simulink model "CM670A_HwAg1Meas"  (R2013b)
settings: Solver=FixedStepDiscrete  SolverMode=SingleTasking  StartTime=0.0  StopTime=22  FixedStep=0.002  RelTol=1e-3
values from neighbouring files (symbols this model uses):
  ELECGLBPRM_DEGPERREV_DEGPERREV_F32 = DataDict.Constant    [CM670A_HwAg1Meas_DataDict.m]
  ELECGLBPRM_HWAGCENTROFFS_HWDEG_F32 = DataDict.Constant    [CM670A_HwAg1Meas_DataDict.m]
  ELECGLBPRM_HWAGSATNLOWRLIM_HWDEG_F32 = DataDict.Constant    [CM670A_HwAg1Meas_DataDict.m]
  ELECGLBPRM_HWAGSATNUPPRLIM_HWDEG_F32 = DataDict.Constant    [CM670A_HwAg1Meas_DataDict.m]
  ELECGLBPRM_HWAGSCA_ULS_F32 = DataDict.Constant    [CM670A_HwAg1Meas_DataDict.m]
  ELECGLBPRM_HWAGSPURGEARRAT_ULS_F32 = DataDict.Constant    [CM670A_HwAg1Meas_DataDict.m]
  ELECGLBPRM_HWAGSPURTORINGGEARRATSNSR0_ULS_F32 = DataDict.Constant    [CM670A_HwAg1Meas_DataDict.m]
  ELECGLBPRM_HWAGSPURTORINGGEARRATSNSR1_ULS_F32 = DataDict.Constant    [CM670A_HwAg1Meas_DataDict.m]
  ELECGLBPRM_NOFLT_CNT_U08 = DataDict.Constant    [CM670A_HwAg1Meas_DataDict.m]
  ELECGLBPRM_OFFSTRIMNOTPRFMD_CNT_U08 = DataDict.Constant    [CM670A_HwAg1Meas_DataDict.m]
  ELECGLBPRM_PRTCLFLT_CNT_U08 = DataDict.Constant    [CM670A_HwAg1Meas_DataDict.m]
  ELECGLBPRM_SKIPSTEPFLT_CNT_U08 = DataDict.Constant    [CM670A_HwAg1Meas_DataDict.m]
  ELECGLBPRM_SNSRINTFLT_CNT_U08 = DataDict.Constant    [CM670A_HwAg1Meas_DataDict.m]
  ELECGLBPRM_VRNRERRFLT_CNT_U08 = DataDict.Constant    [CM670A_HwAg1Meas_DataDict.m]
  HWAG10THTOOTHTRIG_CNT_U08 = DataDict.ConfigParam    [CM670A_HwAg1Meas_DataDict.m]
  HWAG11THTOOTHTRIG_CNT_U08 = DataDict.ConfigParam    [CM670A_HwAg1Meas_DataDict.m]
  HwAg1IfFlt = DataDict.NTC    [CM670A_HwAg1Meas_DataDict.m]
  HwAg1MeasHwAg1IfFltFailStep = DataDict.Calibration    [CM670A_HwAg1Meas_DataDict.m]
  HwAg1MeasHwAg1IfFltPassStep = DataDict.Calibration    [CM670A_HwAg1Meas_DataDict.m]
  HwAg1MeasHwAg1Snsr0PrtclFltFailStep = DataDict.Calibration    [CM670A_HwAg1Meas_DataDict.m]
  HwAg1MeasHwAg1Snsr0PrtclFltPassStep = DataDict.Calibration    [CM670A_HwAg1Meas_DataDict.m]
  HwAg1MeasHwAg1Snsr1PrtclFltFailStep = DataDict.Calibration    [CM670A_HwAg1Meas_DataDict.m]
  HwAg1MeasHwAg1Snsr1PrtclFltPassStep = DataDict.Calibration    [CM670A_HwAg1Meas_DataDict.m]
  HwAg1MeasSnsr0Rev = DataDict.Calibration    [CM670A_HwAg1Meas_DataDict.m]
  HwAg1MeasSnsr1Rev = DataDict.Calibration    [CM670A_HwAg1Meas_DataDict.m]
  HwAg1MeasStep = DataDict.Calibration    [CM670A_HwAg1Meas_DataDict.m]
  HwAg1MeasVrnrErrThd = DataDict.Calibration    [CM670A_HwAg1Meas_DataDict.m]
  HwAg1MfgFlt = DataDict.NTC    [CM670A_HwAg1Meas_DataDict.m]
  HwAg1Snsr0PrtclFlt = DataDict.NTC    [CM670A_HwAg1Meas_DataDict.m]
  HwAg1Snsr1PrtclFlt = DataDict.NTC    [CM670A_HwAg1Meas_DataDict.m]
undefined symbols (not defined in the file or in its folder): NtcSts1, sigbuilder_block, SigQlfr1
libraries: simulink x30, NxtrNvM x3
(part 1 of 5)
settings Model: CovMetricSettings=dcmtrzoiw  CovFilter=CM670A_HwAg1Meas_covfilter  CovHTMLOptions=-sRT=1 -aTS=1 -bRG=1 -bTC=1 -hTR=0 -nFC=0 -scm=1 -bcm=1 -xEv=0  CovModelRefEnable=off  Creator=CZ68DS  LastModifiedBy=CZ68DS
settings SolverCC: PositivePriorityOrder=on  AutoInsertRateTranBlk=on  InsertRTBMode=Always
settings DataIOCC: LimitDataPoints=off  SaveFormat=Structure  ReturnWorkspaceOutputs=on
settings OptimizationCC: InlineParams=on  InlineInvariantSignals=on  PassReuseOutputArgsAs=Individual arguments  ZeroExternalMemoryAtStartup=off  ZeroInternalMemoryAtStartup=off  EfficientFloat2IntCast=on  OptimizeModelRefInitCode=on  LifeSpan=1
settings DebuggingCC: SignalInfNanChecking=error  ReadBeforeWriteMsg=EnableAllAsWarning  WriteAfterWriteMsg=EnableAllAsWarning  WriteAfterReadMsg=EnableAllAsWarning  UnderspecifiedInitializationDetection=Simplified  MergeDetectMultiDrivingBlocksExec=error  SolverPrmCheckMsg=error  InheritedTsInSrcMsg=error  MultiTaskDSMMsg=warning  SingleTaskRateTransMsg=error  TasksWithSamePriorityMsg=error  SigSpecEnsureSampleTimeMsg=error  CheckMatrixSingularityMsg=error  ParameterUnderflowMsg=error  ParameterPrecisionLossMsg=error  ParameterTunabilityLossMsg=error  FixptConstUnderflowMsg=warning  FixptConstOverflowMsg=warning  FixptConstPrecisionLossMsg=warning  VectorMatrixConversionMsg=error  SignalLabelMismatchMsg=error  UnconnectedInputMsg=error  UnconnectedOutputMsg=error  UnconnectedLineMsg=error  SFcnCompatibilityMsg=error  FrameProcessingCompatibilityMsg=error  UniqueDataStoreMsg=warning  BusObjectLabelMismatch=error  RootOutportRequireBusObject=error  AssertControl=DisableAll  ModelReferenceIOMsg=error  ModelReferenceVersionMismatchMessage=warning  ModelReferenceIOMismatchMessage=error  ModelReferenceDataLoggingMessage=error  StateNameClashWarn=warning  StrictBusMsg=ErrorOnBusTreatedAsVector  NonBusSignalsTreatedAsBus=error  SFUnexpectedBacktrackingDiag=error  SFInvalidInputDataAccessInChartInitDiag=error  SFNoUnconditionalDefaultTransitionDiag=error  SFTransitionOutsideNaturalParentDiag=error  SFUnconditionalTransitionShadowingDiag=error  SFUndirectedBroadcastEventsDiag=error
settings HardwareCC: ProdEndianess=LittleEndian  ProdHWDeviceType=Texas Instruments->TMS470
settings ModelReferenceCC: ModelReferenceNumInstancesAllowed=Single
settings RTWCC: SystemTargetFile=autosar.tlc  GenCodeOnly=on  TemplateMakefile=ert_default_tmf  Description=AUTOSAR  GenerateReport=on  ProcessScript=autosar_make_rtw_hook  LaunchReport=on
settings CodeAppCC: GenerateComments=off  IgnoreCustomStorageClasses=off  IgnoreTestpoints=on  CustomSymbolStrType=$N$R$M  CustomSymbolStrBlkIO=$N$M  SimulinkBlockComments=off
settings STFCustomTargetCC: CodeReplacementLibrary=C89/C90 (ANSI)  ParMdlRefBuildCompliant=on  CompOptLevelCompliant=on  IncludeMdlTerminateFcn=off  CombineOutputUpdateFcns=on  SuppressErrorStatus=on  ERTFirstTimeCompliant=on  ERTCustomFileBanners=on  SupportNonFinite=off  SupportComplex=off  SupportContinuousTime=off  SupportNonInlinedSFcns=off  MATLABClassNameForMDSCustomization=Simulink.SoftwareTarget.ERTCustomization  AutosarCompliant=on  GRTInterface=off  SystemTargetFile=autosar.tlc
settings ERTTargetCC: CodeReplacementLibrary=C89/C90 (ANSI)  ConcurrentExecutionCompliant=off  IncludeMdlTerminateFcn=off  SuppressErrorStatus=on  SupportNonFinite=off  SupportComplex=off  ModelStepFunctionPrototypeControlCompliant=off  CPPClassGenCompliant=off  AutosarCompliant=on  InlinedParameterPlacement=NonHierarchical  ERTCustomFileTemplate=example_file_process.tlc  EnableUserReplacementTypes=on

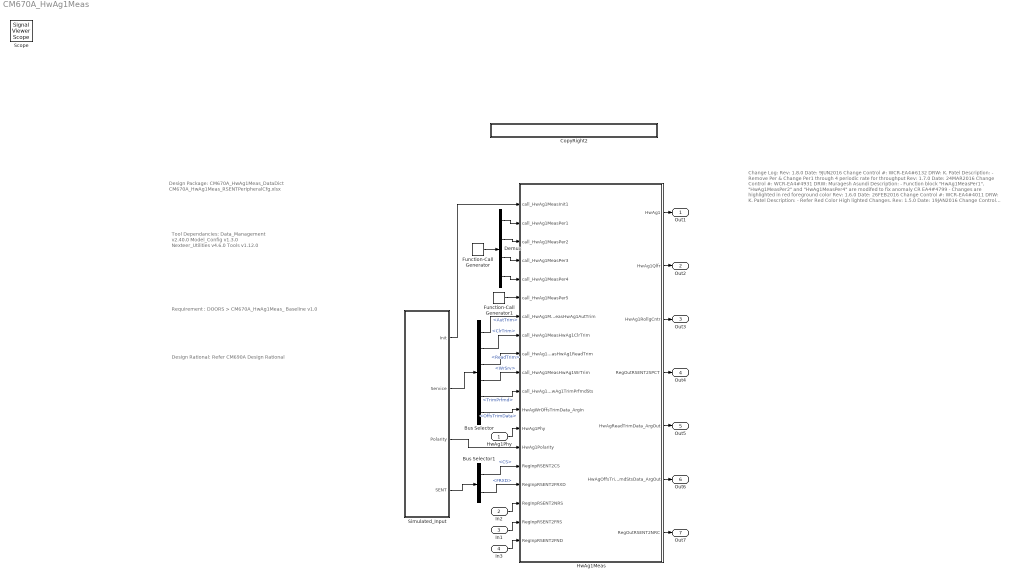
== system CM670A_HwAg1Meas ==
  note: Tool Dependancies:
      |
      | Data_Management v2.40.0
      | Model_Config v1.3.0
      | Nexteer_Utilities v4.6.0
      | Tools v1.12.0
  note: Design Package:
      |
      | CM670A_HwAg1Meas_DataDict
      | CM670A_HwAg1Meas_RSENTPeripheralCfg.xlsx
  note: Requirement :
      |
      | DOORS > CM670A_HwAg1Meas_ Baseline v1.0
  note: Change Log:
      |
      | Rev: 1.8.0
      | Date: 9JUN2016
      | Change Control #: WCR-EA4#6132
      | DRW: K. Patel
      | Description:
      | - Remove Per & Change Per1 through 4 periodic rate for throughput
      |
      |
      | Rev: 1.7.0
      | Date: 24MAR2016
      | Change Control #: WCR-EA4#4931
      | DRW: Muragesh Asundi
      | Description:
      | - Function block "HwAg1MeasPer1", "HwAg1MeasPer2" and "HwAg1MeasPer4" are modifed
      |   to fix anomaly CR EA4#4799
      | - Changes are highlighted in red foreground color
      |
      | Rev: 1.6.0
      | Date: 26FEB2016
      | Change Control #: WCR-EA4#4011
      | DRW: K. Patel
      | Description:
      | - Refer Red Color High lighted Changes.
      |
      | Rev: 1.5.0
      | Date: 19JAN2016
      | Change Control #: WCR-EA4#3382
      | DRW: K. Patel
      | Description:
      | - Refer Red Color High lighted Changes.
      | - "CM670A_HwAg1Meas_RSENTPeripheralCfg.xlsx" change
      | - m file change
      |
      | Rev: 1.4.0
      | Date: 02DEC2015
      | Change Control #: WCR-EA4#2679 Anomaly Fix
      | DRW: K. Patel
      | Description:
      | - Refer Red Color High lighted Changes.
      |
      | Rev: 1.3.0
      | Date: 06OCT2015
      | Change Control #: WCR-EA4#1873, Anomaly:EA4#1856
      | DRW: K. Patel
      | Description:
      | - Skip step Interface fault
      |
      | Rev: 1.2.0
      | Date: 8SEPT2015
      | Change Control #: WCR-EA4#1530, Anomaly:EA4#1354, Anomaly:EA4#1508
      | DRW: K. Patel
      | Description:
      | - Reading Nibble Fix (peripheral register configuration change)
      | - Cleaning CS register before SPCT
      | - Sensor Synchronization logic added
      |
      | Rev: 1.1.0
      | Date: 11AUG2015
      | Change Control #: WCR-EA4#1271
      | DRW: K. Patel
      | Description:
      | - M file correction & Model Correction
      |
      | Rev: 1.0.0
      | Date: 23JUN2015
      | Change Control #: WCR-EA4#910
      | DRW: K. Patel
      | Description:
      | - Initial Release
      |
      | DRW: Keyur Patel
      | Scope:
      | - Model intent to implement EA4 SENT2 based Digital HandWheel Angle implementation for T1xx.
      |    model runs at different function rate:
      |       1) Init - Configure Peripheral
      |       2) 4ms - Per1 & Per2 use for SENT Trigger
      |       3) 4ms - Per3 Read SENT Data from 10 Tooth & Protocol Fault
      |       4) 4ms - Per4 Read SENT Data from 11 Tooth & Protocol Fault
      |       5) 4ms - Per5 Final HwAg calculation
      |       6) 100ms - Per6 Trim Not Performed evaluation
      |       7) Event Trim Service - Auto, Clear, Write, Read, Trim Performed Status
      | - Copyright Blocks added to each layer
  note: Design Rational:
      |
      | Refer CM690A Design Rational
  HwAg1Phy : Inport
  In2 : Inport  Port=2
  In1 : Inport  Port=3
  In3 : Inport  Port=4
  Bus Selector : BusSelector  OutputSignals=AutTrim,ClrTrim,ReadTrim,WrSrv,TrimPrfmd,OffsTrimData
  Bus Selector1 : BusSelector  OutputSignals=CS,FRXD
  CopyRight2 : Subsystem  Description=|  mask(Copyright Information){none=on}
      | Copyright info block.                                               
      |                                                                     
      | Place copyright information at the top of every subsystem in design.
      mask prompts: none "No parameters"
      mask help: Place copyright information at the top of every subsystem in design.
      mask Display:
      | NxtrConf = 'Nexteer Confidential';
      | 
      | sys = bdroot; %handle for the current model ("system")
      | first = get_param(sys,'Created');
      | first = first(end-3:end);  %year is last four digits
      | 
      | last = get_param(sys,'LastModifiedDate');
      | if isempty(last)
      |     last = datestr(now,'yyyy');
      | else
      |     last = last(end-3:end);
      | end
      | 
      | if strcmp(first,last)
      |     fprintf('%s -- Copyright %s Nexteer',NxtrConf,first)
      | else
      |     fprintf('%s -- %s%s- %s Nexteer',NxtrConf,char(169),first,last)
      | end
  Demux : Demux
  Function-Call Generator : simulink/Ports & Subsystems/Function-Call Generator  sample_time=0.002  numberOfIterations=1
      settings: AttributesFormatString=%<sample_time>
  Function-Call Generator1 : simulink/Ports & Subsystems/Function-Call Generator  sample_time=0.100  numberOfIterations=1
  HwAg1Meas : Subsystem  RequirementInfo={} %GIDa_1b511019_32d3_4208_ad3f_5416ab2f5672
  Simulated_Input : Subsystem  Description=Do not Code this block
      settings: AttributesFormatString=%<Description>
  Out1 : Outport
  Out2 : Outport  Port=2
  Out3 : Outport  Port=3
  Out4 : Outport  Port=4
  Out5 : Outport  Port=5
  Out6 : Outport  Port=6
  Out7 : Outport  Port=7
  Scope : SignalViewerScope  IOType=viewer  SampleTime=-1  RefreshTime=0.035000
      settings: YMin=-10  YMax=10
  wires:
  Function-Call Generator/1 -> Demux/1
  HwAg1Meas/1(HwAg1) -> Out1/1
  Demux/1 -> HwAg1Meas/2(call_HwAg1MeasPer1)
  Demux/2 -> HwAg1Meas/3(call_HwAg1MeasPer2)
  Demux/3 -> HwAg1Meas/4(call_HwAg1MeasPer3)
  Function-Call Generator1/1 -> HwAg1Meas/6(call_HwAg1MeasPer5)
  Simulated_Input/3(Polarity) -> HwAg1Meas/14(HwAg1Polarity)
  HwAg1Meas/2(HwAg1Qlfr) -> Out2/1
  HwAg1Meas/3(HwAg1RollgCntr) -> Out3/1
  HwAg1Meas/4(RegOutRSENT2SPCT) -> Out4/1
  HwAg1Meas/5(HwAgReadTrimData_ArgOut) -> Out5/1
  HwAg1Meas/6(HwAgOffsTrimPrfmdStsData_ArgOut) -> Out6/1
  Simulated_Input/2(Service) -> Bus Selector/1
  Bus Selector/1 -> HwAg1Meas/7(call_HwAg1MeasHwAg1AutTrim)  "<AutTrim>"
  Bus Selector/2 -> HwAg1Meas/8(call_HwAg1MeasHwAg1ClrTrim)  "<ClrTrim>"
  Bus Selector/3 -> HwAg1Meas/9(call_HwAg1MeasHwAg1ReadTrim)  "<ReadTrim>"
  Bus Selector/4 -> HwAg1Meas/10(call_HwAg1MeasHwAg1WrTrim)  "<WrSrv>"
  Bus Selector/5 -> HwAg1Meas/11(call_HwAg1MeasHwAg1TrimPrfmdSts)  "<TrimPrfmd>"
  Bus Selector/6 -> HwAg1Meas/12(HwAgWrOffsTrimData_ArgIn)  "<OffsTrimData>"
  Simulated_Input/1(Init) -> HwAg1Meas/1(call_HwAg1MeasInit1)
  HwAg1Phy/1 -> HwAg1Meas/13(HwAg1Phy)
  Simulated_Input/4(SENT) -> Bus Selector1/1
  Bus Selector1/1 -> HwAg1Meas/15(RegInpRSENT2CS)  "<CS>"
  Bus Selector1/2 -> HwAg1Meas/16(RegInpRSENT2FRXD)  "<FRXD>"
  In2/1 -> HwAg1Meas/17(RegInpRSENT2NRS)
  HwAg1Meas/7(RegOutRSENT2NRC) -> Out7/1
  In1/1 -> HwAg1Meas/18(RegInpRSENT2FRS)
  In3/1 -> HwAg1Meas/19(RegInpRSENT2FND)
  Demux/4 -> HwAg1Meas/5(call_HwAg1MeasPer4)

== system CM670A_HwAg1Meas/CopyRight2 ==

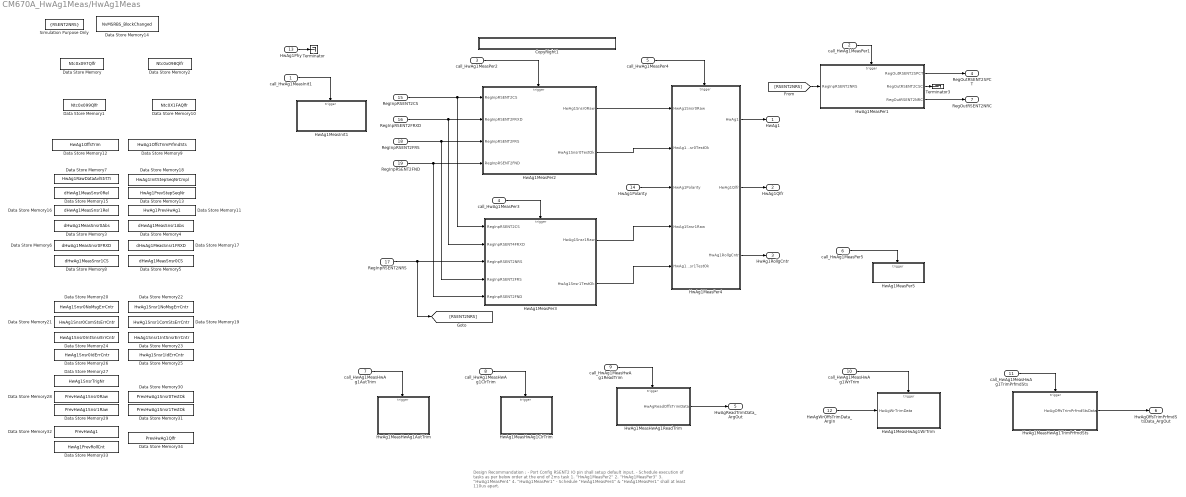
== system CM670A_HwAg1Meas/HwAg1Meas ==
  note: Design Recommandation :
      |
      | - Port Config RSENT2 IO pin shall setup default input.
      | - Schedule execution of tasks as per below order at the end of 2ms task
      |
      |    1.  "HwAg1MeasPer2"
      |    2.  "HwAg1MeasPer3"
      |    3.  "HwAg1MeasPer4"
      |    4.  "HwAg1MeasPer1"
      |
      | - Schedule  "HwAg1MeasPer4" & "HwAg1MeasPer1"  shall at least 110us apart.
  call_HwAg1MeasInit1 : Inport
  call_HwAg1MeasPer1 : Inport  Port=2
      settings: AttributesFormatString=%<SampleTime>
  call_HwAg1MeasPer2 : Inport  Port=3
      settings: AttributesFormatString=%<SampleTime>
  call_HwAg1MeasPer3 : Inport  Port=4
      settings: AttributesFormatString=%<SampleTime>
  call_HwAg1MeasPer4 : Inport  Description=4ms  Port=5
      settings: AttributesFormatString=%<SampleTime>
  call_HwAg1MeasPer5 : Inport  Description=100ms  Port=6
      settings: AttributesFormatString=%<Description>
  call_HwAg1MeasHwAg1AutTrim : Inport  Description=Event  Port=7
      settings: AttributesFormatString=%<Description>
  call_HwAg1MeasHwAg1ClrTrim : Inport  Description=Event  Port=8
      settings: AttributesFormatString=%<Description>
  call_HwAg1MeasHwAg1ReadTrim : Inport  Description=Event  Port=9
      settings: AttributesFormatString=%<Description>
  call_HwAg1MeasHwAg1WrTrim : Inport  Description=Event  Port=10
      settings: AttributesFormatString=%<Description>
  call_HwAg1MeasHwAg1TrimPrfmdSts : Inport  Description=Event  Port=11
      settings: AttributesFormatString=%<Description>
  HwAgWrOffsTrimData_ArgIn : Inport  Port=12
  HwAg1Phy : Inport  Port=13
  HwAg1Polarity : Inport  Port=14  OutDataTypeStr=int8
  RegInpRSENT2CS : Inport  Port=15
  RegInpRSENT2FRXD : Inport  Port=16
  RegInpRSENT2NRS : Inport  Port=17
  RegInpRSENT2FRS : Inport  Port=18
  RegInpRSENT2FND : Inport  Port=19
  CopyRight1 : Subsystem  Description=|  mask(Copyright Information){none=on}
      | Copyright info block.                                               
      |                                                                     
      | Place copyright information at the top of every subsystem in design.
      mask prompts: none "No parameters"
      mask help: Place copyright information at the top of every subsystem in design.
      mask Display:
      | NxtrConf = 'Nexteer Confidential';
      | 
      | sys = bdroot; %handle for the current model ("system")
      | first = get_param(sys,'Created');
      | first = first(end-3:end);  %year is last four digits
      | 
      | last = get_param(sys,'LastModifiedDate');
      | if isempty(last)
      |     last = datestr(now,'yyyy');
      | else
      |     last = last(end-3:end);
      | end
      | 
      | if strcmp(first,last)
      |     fprintf('%s -- Copyright %s Nexteer',NxtrConf,first)
      | else
      |     fprintf('%s -- %s%s- %s Nexteer',NxtrConf,char(169),first,last)
      | end
  Data Store Memory11 : DataStoreMemory  DataStoreName=HwAg1PrevHwAg1  ReadBeforeWriteMsg=warning  WriteAfterWriteMsg=warning  WriteAfterReadMsg=warning  StateMustResolveToSignalObject=on
  Data Store Memory12 : DataStoreMemory  DataStoreName=HwAg1OffsTrim  ReadBeforeWriteMsg=warning  WriteAfterWriteMsg=warning  WriteAfterReadMsg=warning
  Data Store Memory13 : DataStoreMemory  DataStoreName=HwAg1PrevStepSeqNr  ReadBeforeWriteMsg=warning  WriteAfterWriteMsg=warning  WriteAfterReadMsg=warning  StateMustResolveToSignalObject=on
  Data Store Memory14 : DataStoreMemory  Description=|  DataStoreName=NvMSRBS_BlockChanged  ReadBeforeWriteMsg=warning  WriteAfterWriteMsg=warning  WriteAfterReadMsg=warning
      | Simulation Purpose Only.
      | Do Not Code this block
      | NVM Manager Owns this requirement
      settings: AttributesFormatString=%<Description>
  Data Store Memory15 : DataStoreMemory  DataStoreName=dHwAg1MeasSnsr0Rel  ReadBeforeWriteMsg=warning  WriteAfterWriteMsg=warning  WriteAfterReadMsg=warning  StateMustResolveToSignalObject=on
  Data Store Memory16 : DataStoreMemory  DataStoreName=dHwAg1MeasSnsr1Rel  ReadBeforeWriteMsg=warning  WriteAfterWriteMsg=warning  WriteAfterReadMsg=warning  StateMustResolveToSignalObject=on
  Data Store Memory17 : DataStoreMemory  DataStoreName=dHwAg1MeasSnsr1FRXD  ReadBeforeWriteMsg=warning  WriteAfterWriteMsg=warning  WriteAfterReadMsg=warning  StateMustResolveToSignalObject=on
  Data Store Memory18 : DataStoreMemory  DataStoreName=HwAg1InitStepSeqNrCmpl  ReadBeforeWriteMsg=warning  WriteAfterWriteMsg=warning  WriteAfterReadMsg=warning  StateMustResolveToSignalObject=on
  Data Store Memory19 : DataStoreMemory  DataStoreName=HwAg1Snsr1ComStsErrCntr  ReadBeforeWriteMsg=warning  WriteAfterWriteMsg=warning  WriteAfterReadMsg=warning  StateMustResolveToSignalObject=on
  Data Store Memory20 : DataStoreMemory  DataStoreName=HwAg1Snsr0NoMsgErrCntr  ReadBeforeWriteMsg=warning  WriteAfterWriteMsg=warning  WriteAfterReadMsg=warning  StateMustResolveToSignalObject=on
  Data Store Memory21 : DataStoreMemory  DataStoreName=HwAg1Snsr0ComStsErrCntr  ReadBeforeWriteMsg=warning  WriteAfterWriteMsg=warning  WriteAfterReadMsg=warning  StateMustResolveToSignalObject=on
  Data Store Memory22 : DataStoreMemory  DataStoreName=HwAg1Snsr1NoMsgErrCntr  ReadBeforeWriteMsg=warning  WriteAfterWriteMsg=warning  WriteAfterReadMsg=warning  StateMustResolveToSignalObject=on
  Data Store Memory23 : DataStoreMemory  DataStoreName=HwAg1Snsr1IntSnsrErrCntr  ReadBeforeWriteMsg=warning  WriteAfterWriteMsg=warning  WriteAfterReadMsg=warning  StateMustResolveToSignalObject=on
  Data Store Memory24 : DataStoreMemory  DataStoreName=HwAg1Snsr0IntSnsrErrCntr  ReadBeforeWriteMsg=warning  WriteAfterWriteMsg=warning  WriteAfterReadMsg=warning  StateMustResolveToSignalObject=on
  Data Store Memory25 : DataStoreMemory  DataStoreName=HwAg1Snsr1IdErrCntr  ReadBeforeWriteMsg=warning  WriteAfterWriteMsg=warning  WriteAfterReadMsg=warning  StateMustResolveToSignalObject=on
  Data Store Memory26 : DataStoreMemory  DataStoreName=HwAg1Snsr0IdErrCntr  ReadBeforeWriteMsg=warning  WriteAfterWriteMsg=warning  WriteAfterReadMsg=warning  StateMustResolveToSignalObject=on
  Data Store Memory27 : DataStoreMemory  DataStoreName=HwAg1SnsrTrigNr  ReadBeforeWriteMsg=warning  WriteAfterWriteMsg=warning  WriteAfterReadMsg=warning  StateMustResolveToSignalObject=on
  Data Store Memory28 : DataStoreMemory  DataStoreName=PrevHwAg1Snsr0Raw  ReadBeforeWriteMsg=warning  WriteAfterWriteMsg=warning  WriteAfterReadMsg=warning  StateMustResolveToSignalObject=on
  Data Store Memory29 : DataStoreMemory  DataStoreName=PrevHwAg1Snsr1Raw  ReadBeforeWriteMsg=warning  WriteAfterWriteMsg=warning  WriteAfterReadMsg=warning  StateMustResolveToSignalObject=on
  Data Store Memory3 : DataStoreMemory  DataStoreName=dHwAg1MeasSnsr0Abs  ReadBeforeWriteMsg=warning  WriteAfterWriteMsg=warning  WriteAfterReadMsg=warning  StateMustResolveToSignalObject=on
  Data Store Memory30 : DataStoreMemory  DataStoreName=PrevHwAg1Snsr0TestOk  ReadBeforeWriteMsg=warning  WriteAfterWriteMsg=warning  WriteAfterReadMsg=warning  StateMustResolveToSignalObject=on
  Data Store Memory31 : DataStoreMemory  DataStoreName=PrevHwAg1Snsr1TestOk  ReadBeforeWriteMsg=warning  WriteAfterWriteMsg=warning  WriteAfterReadMsg=warning  StateMustResolveToSignalObject=on
  Data Store Memory32 : DataStoreMemory  DataStoreName=PrevHwAg1  ReadBeforeWriteMsg=warning  WriteAfterWriteMsg=warning  WriteAfterReadMsg=warning  StateMustResolveToSignalObject=on
  Data Store Memory33 : DataStoreMemory  DataStoreName=HwAg1PrevRollCnt  ReadBeforeWriteMsg=warning  WriteAfterWriteMsg=warning  WriteAfterReadMsg=warning  StateMustResolveToSignalObject=on
  Data Store Memory34 : DataStoreMemory  DataStoreName=PrevHwAg1Qlfr  ReadBeforeWriteMsg=warning  WriteAfterWriteMsg=warning  WriteAfterReadMsg=warning  InitialValue=SigQlfr1.SIGQLFR_NORES  OutDataTypeStr=Enum: SigQlfr1  StateMustResolveToSignalObject=on
  Data Store Memory4 : DataStoreMemory  DataStoreName=dHwAg1MeasSnsr1Abs  ReadBeforeWriteMsg=warning  WriteAfterWriteMsg=warning  WriteAfterReadMsg=warning  StateMustResolveToSignalObject=on
  Data Store Memory5 : DataStoreMemory  DataStoreName=dHwAg1MeasSnsr0CS  ReadBeforeWriteMsg=warning  WriteAfterWriteMsg=warning  WriteAfterReadMsg=warning  StateMustResolveToSignalObject=on
  Data Store Memory6 : DataStoreMemory  DataStoreName=dHwAg1MeasSnsr0FRXD  ReadBeforeWriteMsg=warning  WriteAfterWriteMsg=warning  WriteAfterReadMsg=warning  StateMustResolveToSignalObject=on
  Data Store Memory7 : DataStoreMemory  DataStoreName=HwAg1RawDataAvlStrtTi  ReadBeforeWriteMsg=warning  WriteAfterWriteMsg=warning  WriteAfterReadMsg=warning  StateMustResolveToSignalObject=on
  Data Store Memory8 : DataStoreMemory  DataStoreName=dHwAg1MeasSnsr1CS  ReadBeforeWriteMsg=warning  WriteAfterWriteMsg=warning  WriteAfterReadMsg=warning  StateMustResolveToSignalObject=on
  Data Store Memory9 : DataStoreMemory  DataStoreName=HwAg1OffsTrimPrfmdSts  ReadBeforeWriteMsg=warning  WriteAfterWriteMsg=warning  WriteAfterReadMsg=warning
  Data Store Memory : DataStoreMemory  DataStoreName=Ntc0x097Qlfr  ReadBeforeWriteMsg=warning  WriteAfterWriteMsg=warning  WriteAfterReadMsg=warning  OutDataTypeStr=uint8
      settings: AttributesFormatString=|
      | Simulation Purpose Only.
      | Do Not Code this block
      | Diagnostic Manager Owns this requirement
  Data Store Memory1 : DataStoreMemory  DataStoreName=Ntc0x099Qlfr  ReadBeforeWriteMsg=warning  WriteAfterWriteMsg=warning  WriteAfterReadMsg=warning  OutDataTypeStr=uint8
      settings: AttributesFormatString=|
      | Simulation Purpose Only.
      | Do Not Code this block
      | Diagnostic Manager Owns this requirement
  Data Store Memory10 : DataStoreMemory  DataStoreName=Ntc0X1FAQlfr  ReadBeforeWriteMsg=warning  WriteAfterWriteMsg=warning  WriteAfterReadMsg=warning  OutDataTypeStr=uint8
      settings: AttributesFormatString=|
      | Simulation Purpose Only.
      | Do Not Code this block
      | Diagnostic Manager Owns this requirement
  Data Store Memory2 : DataStoreMemory  DataStoreName=Ntc0x098Qlfr  ReadBeforeWriteMsg=warning  WriteAfterWriteMsg=warning  WriteAfterReadMsg=warning  OutDataTypeStr=uint8
      settings: AttributesFormatString=|
      | Simulation Purpose Only.
      | Do Not Code this block
      | Diagnostic Manager Owns this requirement
  HwAg1MeasHwAg1AutTrim : Subsystem  RequirementInfo={'linktype_rmi_doors' '0000cf44 (/ESG Group/FDD Module Requirements/EA4 Specific/CM670A_HwAg1Meas)' '#CM670A_90' 'true' 'REQ: CM670A_90' '' } %GIDa_ea94ffee_6a60_4ad4_8777_fa2e1209d3e2  TreatAsAtomicUnit=on
  HwAg1MeasHwAg1ClrTrim : Subsystem  RequirementInfo={'linktype_rmi_doors' '0000cf44 (/ESG Group/FDD Module Requirements/EA4 Specific/CM670A_HwAg1Meas)' '#CM670A_88' 'true' 'REQ: CM670A_88' '' } %GIDa_ac4d7135_c09e_4b99_819a_ee37d51d6394  TreatAsAtomicUnit=on
  HwAg1MeasHwAg1ReadTrim : Subsystem  RequirementInfo={'linktype_rmi_doors' '0000cf44 (/ESG Group/FDD Module Requirements/EA4 Specific/CM670A_HwAg1Meas)' '#CM670A_86' 'true' 'REQ: CM670A_86' '' } %GIDa_cdad271c_f4aa_4684_91af_0774478ab1dd  TreatAsAtomicUnit=on
  HwAg1MeasHwAg1TrimPrfmdSts : Subsystem  RequirementInfo={'linktype_rmi_doors' '0000cf44 (/ESG Group/FDD Module Requirements/EA4 Specific/CM670A_HwAg1Meas)' '#CM670A_87' 'true' 'REQ: CM670A_87' '' } %GIDa_f9e60140_9f20_40c9_8f6d_edf000506692  TreatAsAtomicUnit=on
  HwAg1MeasHwAg1WrTrim : Subsystem  RequirementInfo={'linktype_rmi_doors' '0000cf44 (/ESG Group/FDD Module Requirements/EA4 Specific/CM670A_HwAg1Meas)' '#CM670A_89' 'true' 'REQ: CM670A_89' '' } %GIDa_3e323fa6_2ebf_495c_adb5_a3e2347a88cc  TreatAsAtomicUnit=on
  HwAg1MeasInit1 : Subsystem  TreatAsAtomicUnit=on
  HwAg1MeasPer1 : Subsystem  RequirementInfo={'linktype_rmi_doors' '0000cf44 (/ESG Group/FDD Module Requirements/EA4 Specific/CM670A_HwAg1Meas)' '#CM670A_53' 'true' 'REQ: CM670A_53' '' } %GIDa_bc322e89_7505_4ced_bd58_d5630035f58c  TreatAsAtomicUnit=on
  HwAg1MeasPer2 : Subsystem  RequirementInfo={'linktype_rmi_doors' '0000cf44 (/ESG Group/FDD Module Requirements/EA4 Specific/CM670A_HwAg1Meas)' '#CM670A_54' 'true' 'REQ: CM670A_54' '' ; 'linktype_rmi_doors' '0000cf44 (/ESG Group/FDD Module Requirements/EA4 Specific/CM670A_HwAg1Meas)' '#CM670A_39' 'true' 'REQ: CM670A_39' '' } %GIDa_9b2c116c_3a4f_439a_af77_b112da5d765b  TreatAsAtomicUnit=on
  HwAg1MeasPer3 : Subsystem  RequirementInfo={'linktype_rmi_doors' '0000cf44 (/ESG Group/FDD Module Requirements/EA4 Specific/CM670A_HwAg1Meas)' '#CM670A_54' 'true' 'REQ: CM670A_54' '' ; 'linktype_rmi_doors' '0000cf44 (/ESG Group/FDD Module Requirements/EA4 Specific/CM670A_HwAg1Meas)' '#CM670A_60' 'true' 'REQ: CM670A_60' '' } %GIDa_7cda62b4_5588_448d_b03e_99bd27827f7d  TreatAsAtomicUnit=on
  HwAg1MeasPer4 : Subsystem  RequirementInfo={'linktype_rmi_doors' '0000cf44 (/ESG Group/FDD Module Requirements/EA4 Specific/CM670A_HwAg1Meas)' '#CM670A_95' 'true' 'REQ: CM670A_95' '' } %GIDa_d2359c71_dfd5_4281_9f6c_59b61df0ca5b  TreatAsAtomicUnit=on
  HwAg1MeasPer5 : Subsystem  RequirementInfo={'linktype_rmi_doors' '0000cf44 (/ESG Group/FDD Module Requirements/EA4 Specific/CM670A_HwAg1Meas)' '#CM670A_80' 'true' 'REQ: CM670A_80' '' } %GIDa_d0a6efa9_4f14_452b_9991_ec4ccddab763  TreatAsAtomicUnit=on
  Simulation Purpose Only : GotoTagVisibility  GotoTag=RSENT2NRS
  Terminator : Terminator
  Terminator3 : Terminator
  HwAg1 : Outport
  HwAg1Qlfr : Outport  Port=2
  HwAg1RollgCntr : Outport  Port=3
  RegOutRSENT2SPCT : Outport  Port=4
  HwAgReadTrimData_ArgOut : Outport  Port=5
  HwAgOffsTrimPrfmdStsData_ArgOut : Outport  Port=6
  RegOutRSENT2NRC : Outport  Port=7
  wires:
  call_HwAg1MeasPer2/1 -> HwAg1MeasPer2/Trigger
  call_HwAg1MeasInit1/1 -> HwAg1MeasInit1/Trigger
  RegInpRSENT2CS/1 -> HwAg1MeasPer3/1(RegInpRSENT2CS), HwAg1MeasPer2/1(RegInpRSENT2CS)
  HwAg1Phy/1 -> Terminator/1
  HwAg1MeasPer4/1(HwAg1) -> HwAg1/1
  HwAg1MeasPer4/2(HwAg1Qlfr) -> HwAg1Qlfr/1
  HwAg1MeasPer4/3(HwAg1RollgCntr) -> HwAg1RollgCntr/1
  call_HwAg1MeasPer3/1 -> HwAg1MeasPer3/Trigger
  call_HwAg1MeasPer4/1 -> HwAg1MeasPer4/Trigger
  HwAg1Polarity/1 -> HwAg1MeasPer4/3(HwAg1Polarity)
  call_HwAg1MeasPer1/1 -> HwAg1MeasPer1/Trigger
  call_HwAg1MeasHwAg1AutTrim/1 -> HwAg1MeasHwAg1AutTrim/Trigger
  call_HwAg1MeasHwAg1ClrTrim/1 -> HwAg1MeasHwAg1ClrTrim/Trigger
  call_HwAg1MeasHwAg1ReadTrim/1 -> HwAg1MeasHwAg1ReadTrim/Trigger
  call_HwAg1MeasHwAg1WrTrim/1 -> HwAg1MeasHwAg1WrTrim/Trigger
  call_HwAg1MeasHwAg1TrimPrfmdSts/1 -> HwAg1MeasHwAg1TrimPrfmdSts/Trigger
  HwAgWrOffsTrimData_ArgIn/1 -> HwAg1MeasHwAg1WrTrim/1(HwAgWrTrimData)
  HwAg1MeasHwAg1ReadTrim/1(HwAgReadOffsTrimData) -> HwAgReadTrimData_ArgOut/1
  HwAg1MeasHwAg1TrimPrfmdSts/1(HwAgOffsTrimPrfmdStsData) -> HwAgOffsTrimPrfmdStsData_ArgOut/1
  call_HwAg1MeasPer5/1 -> HwAg1MeasPer5/Trigger
  RegInpRSENT2FRXD/1 -> HwAg1MeasPer3/2(RegInpRSENT4FRXD), HwAg1MeasPer2/2(RegInpRSENT2FRXD)
  HwAg1MeasPer2/1(HwAg1Snsr0Raw) -> HwAg1MeasPer4/1(HwAg1Snsr0Raw)
  HwAg1MeasPer2/2(HwAg1Snsr0TestOk) -> HwAg1MeasPer4/2(HwAg1Snsr0TestOk)
  HwAg1MeasPer3/1(HwAg1Snsr1Raw) -> HwAg1MeasPer4/4(HwAg1Snsr1Raw)
  HwAg1MeasPer3/2(HwAg1Snsr1TestOk) -> HwAg1MeasPer4/5(HwAg1Snsr1TestOk)
  RegInpRSENT2NRS/1 -> HwAg1MeasPer3/3(RegInpRSENT2NRS), [RSENT2NRS]
  HwAg1MeasPer1/3(RegOutRSENT2NRC) -> RegOutRSENT2NRC/1
  RegInpRSENT2FRS/1 -> HwAg1MeasPer2/3(RegInpRSENT2FRS), HwAg1MeasPer3/4(RegInpRSENT2FRS)
  RegInpRSENT2FND/1 -> HwAg1MeasPer3/5(RegInpRSENT2FND), HwAg1MeasPer2/4(RegInpRSENT2FND)
  HwAg1MeasPer1/2(RegOutRSENT2CSC) -> Terminator3/1
  [RSENT2NRS] -> HwAg1MeasPer1/1(RegInpRSENT2NRS)
  HwAg1MeasPer1/1(RegOutRSENT2SPCT) -> RegOutRSENT2SPCT/1

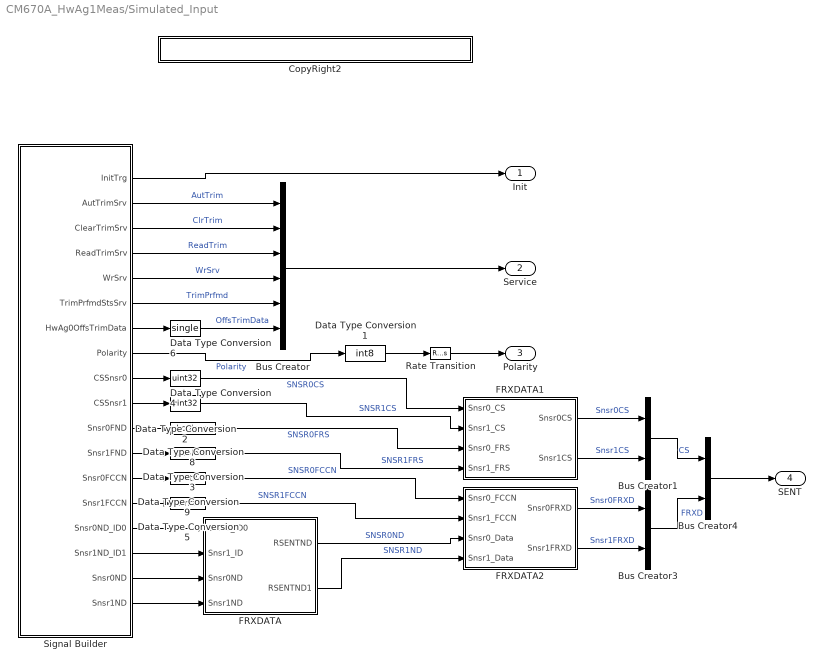
== system CM670A_HwAg1Meas/Simulated_Input ==
  Bus Creator : BusCreator  Inputs=6
  Bus Creator1 : BusCreator  Inputs=2
  Bus Creator3 : BusCreator  Inputs=2
  Bus Creator4 : BusCreator  Inputs=2
  CopyRight2 : Subsystem  Description=|  mask(Copyright Information){none=on}
      | Copyright info block.                                               
      |                                                                     
      | Place copyright information at the top of every subsystem in design.
      mask prompts: none "No parameters"
      mask help: Place copyright information at the top of every subsystem in design.
      mask Display:
      | NxtrConf = 'Nexteer Confidential';
      | 
      | sys = bdroot; %handle for the current model ("system")
      | first = get_param(sys,'Created');
      | first = first(end-3:end);  %year is last four digits
      | 
      | last = get_param(sys,'LastModifiedDate');
      | if isempty(last)
      |     last = datestr(now,'yyyy');
      | else
      |     last = last(end-3:end);
      | end
      | 
      | if strcmp(first,last)
      |     fprintf('%s -- Copyright %s Nexteer',NxtrConf,first)
      | else
      |     fprintf('%s -- %s%s- %s Nexteer',NxtrConf,char(169),first,last)
      | end
  Data Type Conversion1 : DataTypeConversion  OutDataTypeStr=int8
  Data Type Conversion2 : DataTypeConversion  OutDataTypeStr=uint32
  Data Type Conversion3 : DataTypeConversion  OutDataTypeStr=boolean
  Data Type Conversion4 : DataTypeConversion  OutDataTypeStr=uint32
  Data Type Conversion5 : DataTypeConversion  OutDataTypeStr=uint8
  Data Type Conversion6 : DataTypeConversion  OutDataTypeStr=single
  Data Type Conversion8 : DataTypeConversion  OutDataTypeStr=boolean
  Data Type Conversion9 : DataTypeConversion  OutDataTypeStr=uint8
  FRXDATA : Subsystem
  FRXDATA1 : Subsystem
  FRXDATA2 : Subsystem
  Rate Transition : RateTransition
  Signal Builder : Subsystem  Tag=STV Subsys  LoadFcn=sigbuilder_block('load');  StartFcn=sigbuilder_block('start');  StopFcn=sigbuilder_block('stop');  ClipboardFcn=sigbuilder_block('clipboard');  mask(Sigbuilder block){}
      mask help: Simulink:masks:SigbuilderBlock_MD
      mask init:
      | if ~strcmp(get_param(bdroot(gcbh),'SimulationStatus'),'stopped') tuvar = sigbuilder_block('maskInit'); end
      settings: CopyFcn=sigbuilder_block('copy');  DeleteFcn=sigbuilder_block('delete');  ModelCloseFcn=sigbuilder_block('modelClose');  PreSaveFcn=sigbuilder_block('preSave');  PauseFcn=sigbuilder_block('pause');  ContinueFcn=sigbuilder_block('continue');  NameChangeFcn=sigbuilder_block('namechange');  OpenFcn=sigbuilder_block('open',[51 6 967.5 507 ]);  CloseFcn=sigbuilder_block('close');
      mask Display: plot(0, 0, 100, 100,[2, 2, 32, 32, 2], [68, 8, 8, 68, 68],[32, 2], [38, 38], [32, 19, 2],[53, 60, 44], [32, 17, 17, 2],[16, 16, 31, 31]);txt = getActiveGroup(gcbh);text(2, 100, txt,'verticalAlignment', 'top');
  Init : Outport
  Service : Outport  Port=2
  Polarity : Outport  Port=3
  SENT : Outport  Port=4
  wires:
  Signal Builder/8(Polarity) -> Data Type Conversion1/1  "Polarity"
  Signal Builder/1(InitTrg) -> Init/1
  Signal Builder/7(HwAg0OffsTrimData) -> Data Type Conversion6/1
  Signal Builder/6(TrimPrfmdStsSrv) -> Bus Creator/5  "TrimPrfmd"
  Signal Builder/5(WrSrv) -> Bus Creator/4  "WrSrv"
  Signal Builder/4(ReadTrimSrv) -> Bus Creator/3  "ReadTrim"
  Signal Builder/3(ClearTrimSrv) -> Bus Creator/2  "ClrTrim"
  Signal Builder/2(AutTrimSrv) -> Bus Creator/1  "AutTrim"
  Signal Builder/10(CSSnsr1) -> Data Type Conversion2/1
  Signal Builder/15(Snsr0ND_ID0) -> FRXDATA/1(Snsr0_ID0)
  Signal Builder/16(Snsr1ND_ID1) -> FRXDATA/2(Snsr1_ID)
  Signal Builder/17(Snsr0ND) -> FRXDATA/3(Snsr0ND)
  Signal Builder/9(CSSnsr0) -> Data Type Conversion4/1
  Signal Builder/11(Snsr0FND) -> Data Type Conversion8/1
  Signal Builder/12(Snsr1FND) -> Data Type Conversion3/1
  Signal Builder/13(Snsr0FCCN) -> Data Type Conversion9/1
  Signal Builder/14(Snsr1FCCN) -> Data Type Conversion5/1
  Signal Builder/18(Snsr1ND) -> FRXDATA/4(Snsr1ND)
  Bus Creator/1 -> Service/1
  FRXDATA/1(RSENTND) -> FRXDATA2/3(Snsr0_Data)  "SNSR0ND"
  FRXDATA/2(RSENTND1) -> FRXDATA2/4(Snsr1_Data)  "SNSR1ND"
  Data Type Conversion1/1 -> Rate Transition/1
  Rate Transition/1 -> Polarity/1
  Data Type Conversion4/1 -> FRXDATA1/1(Snsr0_CS)  "SNSR0CS"
  Data Type Conversion2/1 -> FRXDATA1/2(Snsr1_CS)  "SNSR1CS"
  Data Type Conversion8/1 -> FRXDATA1/3(Snsr0_FRS)  "SNSR0FRS"
  Data Type Conversion3/1 -> FRXDATA1/4(Snsr1_FRS)  "SNSR1FRS"
  Data Type Conversion9/1 -> FRXDATA2/1(Snsr0_FCCN)  "SNSR0FCCN"
  Data Type Conversion5/1 -> FRXDATA2/2(Snsr1_FCCN)  "SNSR1FCCN"
  Data Type Conversion6/1 -> Bus Creator/6  "OffsTrimData"
  FRXDATA1/2(Snsr1CS) -> Bus Creator1/2  "Snsr1CS"
  FRXDATA1/1(Snsr0CS) -> Bus Creator1/1  "Snsr0CS"
  FRXDATA2/1(Snsr0FRXD) -> Bus Creator3/1  "Snsr0FRXD"
  FRXDATA2/2(Snsr1FRXD) -> Bus Creator3/2  "Snsr1FRXD"
  Bus Creator1/1 -> Bus Creator4/1  "CS"
  Bus Creator3/1 -> Bus Creator4/2  "FRXD"
  Bus Creator4/1 -> SENT/1

== system CM670A_HwAg1Meas/HwAg1Meas/CopyRight1 ==

== system CM670A_HwAg1Meas/HwAg1Meas/HwAg1MeasHwAg1AutTrim ==
  function : TriggerPort
  CopyRight2 : Subsystem  Description=|  mask(Copyright Information){none=on}
      | Copyright info block.                                               
      |                                                                     
      | Place copyright information at the top of every subsystem in design.
      mask prompts: none "No parameters"
      mask help: Place copyright information at the top of every subsystem in design.
      mask Display:
      | NxtrConf = 'Nexteer Confidential';
      | 
      | sys = bdroot; %handle for the current model ("system")
      | first = get_param(sys,'Created');
      | first = first(end-3:end);  %year is last four digits
      | 
      | last = get_param(sys,'LastModifiedDate');
      | if isempty(last)
      |     last = datestr(now,'yyyy');
      | else
      |     last = last(end-3:end);
      | end
      | 
      | if strcmp(first,last)
      |     fprintf('%s -- Copyright %s Nexteer',NxtrConf,first)
      | else
      |     fprintf('%s -- %s%s- %s Nexteer',NxtrConf,char(169),first,last)
      | end
  NVM Shadow RAM : DataStoreWrite  RequirementInfo={'linktype_rmi_doors' '0000cf44 (/ESG Group/FDD Module Requirements/EA4 Specific/CM670A_HwAg1Meas)' '#CM670A_86' 'true' 'REQ: CM670A_86' '' } %GIDa_c48bf4d8_e676_4fba_a351_533fe7cd0c6e  DataStoreName=HwAg1OffsTrim
  NVM1 Shadow RAM : DataStoreWrite  RequirementInfo={'linktype_rmi_doors' '0000cf44 (/ESG Group/FDD Module Requirements/EA4 Specific/CM670A_HwAg1Meas)' '#CM670A_85' 'true' 'REQ: CM670A_85' '' } %GIDa_a97d023e_c210_4163_b9cc_4aaf2b68072e  DataStoreName=HwAg1OffsTrimPrfmdSts
  PIM : DataStoreRead  Priority=10  DataStoreName=HwAg1PrevHwAg1
      settings: AttributesFormatString=Priority=%<Priority>
  Set : Constant
  Set Ram Block Status : NxtrNvM/Set Ram Block Status  FuncName=Set Ram Block Status  NvMBlockName=HwAg1Offs  VoidFuncRtn=on  BlockChanged_DSN=NvMSRBS_BlockChanged  Return_DSN=NvMSRBS_Return
      settings: AttributesFormatString=%<FuncName>
  Set3 : Constant
  wires:
  PIM/1 -> NVM Shadow RAM/1
  Set/1 -> NVM1 Shadow RAM/1
  Set3/1 -> Set Ram Block Status/1

== system CM670A_HwAg1Meas/HwAg1Meas/HwAg1MeasHwAg1ClrTrim ==
  function : TriggerPort
  Clear1 : Constant  Value=0  OutDataTypeStr=single
  Clear2 : Constant  Value=0
  CopyRight2 : Subsystem  Description=|  mask(Copyright Information){none=on}
      | Copyright info block.                                               
      |                                                                     
      | Place copyright information at the top of every subsystem in design.
      mask prompts: none "No parameters"
      mask help: Place copyright information at the top of every subsystem in design.
      mask Display:
      | NxtrConf = 'Nexteer Confidential';
      | 
      | sys = bdroot; %handle for the current model ("system")
      | first = get_param(sys,'Created');
      | first = first(end-3:end);  %year is last four digits
      | 
      | last = get_param(sys,'LastModifiedDate');
      | if isempty(last)
      |     last = datestr(now,'yyyy');
      | else
      |     last = last(end-3:end);
      | end
      | 
      | if strcmp(first,last)
      |     fprintf('%s -- Copyright %s Nexteer',NxtrConf,first)
      | else
      |     fprintf('%s -- %s%s- %s Nexteer',NxtrConf,char(169),first,last)
      | end
  NVM Shadow RAM : DataStoreWrite  RequirementInfo={'linktype_rmi_doors' '0000cf44 (/ESG Group/FDD Module Requirements/EA4 Specific/CM670A_HwAg1Meas)' '#CM670A_86' 'true' 'REQ: CM670A_86' '' } %GIDa_8ccce71d_7994_42b7_8f38_740ca71fc321  DataStoreName=HwAg1OffsTrim
  NVM1 Shadow RAM : DataStoreWrite  RequirementInfo={'linktype_rmi_doors' '0000cf44 (/ESG Group/FDD Module Requirements/EA4 Specific/CM670A_HwAg1Meas)' '#CM670A_85' 'true' 'REQ: CM670A_85' '' } %GIDa_d7bc93a5_b812_40ff_9390_fa70717297a5  DataStoreName=HwAg1OffsTrimPrfmdSts
  Set Ram Block Status : NxtrNvM/Set Ram Block Status  FuncName=Set Ram Block Status  NvMBlockName=HwAg1Offs  VoidFuncRtn=on  BlockChanged_DSN=NvMSRBS_BlockChanged  Return_DSN=NvMSRBS_Return
      settings: AttributesFormatString=%<FuncName>
  Set3 : Constant
  wires:
  Clear1/1 -> NVM Shadow RAM/1
  Clear2/1 -> NVM1 Shadow RAM/1
  Set3/1 -> Set Ram Block Status/1

== system CM670A_HwAg1Meas/HwAg1Meas/HwAg1MeasHwAg1ReadTrim ==
  function : TriggerPort
  CopyRight2 : Subsystem  Description=|  mask(Copyright Information){none=on}
      | Copyright info block.                                               
      |                                                                     
      | Place copyright information at the top of every subsystem in design.
      mask prompts: none "No parameters"
      mask help: Place copyright information at the top of every subsystem in design.
      mask Display:
      | NxtrConf = 'Nexteer Confidential';
      | 
      | sys = bdroot; %handle for the current model ("system")
      | first = get_param(sys,'Created');
      | first = first(end-3:end);  %year is last four digits
      | 
      | last = get_param(sys,'LastModifiedDate');
      | if isempty(last)
      |     last = datestr(now,'yyyy');
      | else
      |     last = last(end-3:end);
      | end
      | 
      | if strcmp(first,last)
      |     fprintf('%s -- Copyright %s Nexteer',NxtrConf,first)
      | else
      |     fprintf('%s -- %s%s- %s Nexteer',NxtrConf,char(169),first,last)
      | end
  NVM Shadow RAM : DataStoreRead  DataStoreName=HwAg1OffsTrim
  HwAgReadOffsTrimData : Outport
  wires:
  NVM Shadow RAM/1 -> HwAgReadOffsTrimData/1

== system CM670A_HwAg1Meas/HwAg1Meas/HwAg1MeasHwAg1TrimPrfmdSts ==
  function : TriggerPort
  CopyRight2 : Subsystem  Description=|  mask(Copyright Information){none=on}
      | Copyright info block.                                               
      |                                                                     
      | Place copyright information at the top of every subsystem in design.
      mask prompts: none "No parameters"
      mask help: Place copyright information at the top of every subsystem in design.
      mask Display:
      | NxtrConf = 'Nexteer Confidential';
      | 
      | sys = bdroot; %handle for the current model ("system")
      | first = get_param(sys,'Created');
      | first = first(end-3:end);  %year is last four digits
      | 
      | last = get_param(sys,'LastModifiedDate');
      | if isempty(last)
      |     last = datestr(now,'yyyy');
      | else
      |     last = last(end-3:end);
      | end
      | 
      | if strcmp(first,last)
      |     fprintf('%s -- Copyright %s Nexteer',NxtrConf,first)
      | else
      |     fprintf('%s -- %s%s- %s Nexteer',NxtrConf,char(169),first,last)
      | end
  Data Store Read1 : DataStoreRead  DataStoreName=HwAg1OffsTrimPrfmdSts
  HwAgOffsTrimPrfmdStsData : Outport
  wires:
  Data Store Read1/1 -> HwAgOffsTrimPrfmdStsData/1

== system CM670A_HwAg1Meas/HwAg1Meas/HwAg1MeasHwAg1WrTrim ==
  HwAgWrTrimData : Inport
  function : TriggerPort
  CopyRight2 : Subsystem  Description=|  mask(Copyright Information){none=on}
      | Copyright info block.                                               
      |                                                                     
      | Place copyright information at the top of every subsystem in design.
      mask prompts: none "No parameters"
      mask help: Place copyright information at the top of every subsystem in design.
      mask Display:
      | NxtrConf = 'Nexteer Confidential';
      | 
      | sys = bdroot; %handle for the current model ("system")
      | first = get_param(sys,'Created');
      | first = first(end-3:end);  %year is last four digits
      | 
      | last = get_param(sys,'LastModifiedDate');
      | if isempty(last)
      |     last = datestr(now,'yyyy');
      | else
      |     last = last(end-3:end);
      | end
      | 
      | if strcmp(first,last)
      |     fprintf('%s -- Copyright %s Nexteer',NxtrConf,first)
      | else
      |     fprintf('%s -- %s%s- %s Nexteer',NxtrConf,char(169),first,last)
      | end
  NVM Shadow RAM : DataStoreWrite  RequirementInfo={'linktype_rmi_doors' '0000cf44 (/ESG Group/FDD Module Requirements/EA4 Specific/CM670A_HwAg1Meas)' '#CM670A_86' 'true' 'REQ: CM670A_86' '' } %GIDa_dfafe5ae_08bd_4bd9_b83d_678516e8f399  DataStoreName=HwAg1OffsTrim
  NVM1 Shadow RAM : DataStoreWrite  RequirementInfo={'linktype_rmi_doors' '0000cf44 (/ESG Group/FDD Module Requirements/EA4 Specific/CM670A_HwAg1Meas)' '#CM670A_85' 'true' 'REQ: CM670A_85' '' } %GIDa_43ae7be7_0f33_49ca_abd0_4c14044b69a7  DataStoreName=HwAg1OffsTrimPrfmdSts
  Set : Constant
  Set Ram Block Status : NxtrNvM/Set Ram Block Status  FuncName=Set Ram Block Status  NvMBlockName=HwAg1Offs  VoidFuncRtn=on  BlockChanged_DSN=NvMSRBS_BlockChanged  Return_DSN=NvMSRBS_Return
      settings: AttributesFormatString=%<FuncName>
  Set3 : Constant
  wires:
  Set/1 -> NVM1 Shadow RAM/1
  HwAgWrTrimData/1 -> NVM Shadow RAM/1
  Set3/1 -> Set Ram Block Status/1

== system CM670A_HwAg1Meas/HwAg1Meas/HwAg1MeasInit1 ==
  note: Follow below steps in same order:
      |
      | 1. Enable Configuration mode, RSENT2MDC.OMC = 1U
      | 2. Verify whether peripheral is in Configuration mode RSENT2MST.OMS ==1U and wait till 2us*, it is in configuration mode
      | 3. Configure the SENT Register as per  "CM670A_HwAg1Meas_RSENTPeripheralCfg.xlsx"
      | 4. Enable Operation active mode, RSENT2MDC.OMC = 5U
      | 5. Verify whether peripheral is in Opertation active mode RSENT2MST.OMS ==5U and wait till 2us* , it is in Opertation active mode
      | 6. Client Call "IoHwAb_SetFctPrphlHwAg1"- Port Configuration shall change to output in alternate mode from default input for RSENT2 SPCO IO pin.
      |
      | Note: * - actual minimum is 150ns as per Scott Winder email from Renesas
  function : TriggerPort  TriggerType=falling
  CopyRight2 : Subsystem  Description=|  mask(Copyright Information){none=on}
      | Copyright info block.                                               
      |                                                                     
      | Place copyright information at the top of every subsystem in design.
      mask prompts: none "No parameters"
      mask help: Place copyright information at the top of every subsystem in design.
      mask Display:
      | NxtrConf = 'Nexteer Confidential';
      | 
      | sys = bdroot; %handle for the current model ("system")
      | first = get_param(sys,'Created');
      | first = first(end-3:end);  %year is last four digits
      | 
      | last = get_param(sys,'LastModifiedDate');
      | if isempty(last)
      |     last = datestr(now,'yyyy');
      | else
      |     last = last(end-3:end);
      | end
      | 
      | if strcmp(first,last)
      |     fprintf('%s -- Copyright %s Nexteer',NxtrConf,first)
      | else
      |     fprintf('%s -- %s%s- %s Nexteer',NxtrConf,char(169),first,last)
      | end
  GetRefTmr1MicroSec32bit : Subsystem
      settings: AttributesFormatString=Client Call : Start Time
  GetTiSpan1MicroSec32bit : Subsystem
  IoHwAb_SetFctPrphlHwAg1 : Subsystem
  Terminator1 : Terminator
  wires:
  GetRefTmr1MicroSec32bit/1(RefTmr) -> GetTiSpan1MicroSec32bit/1(RefTmr)
  GetTiSpan1MicroSec32bit/1(TiSpan) -> Terminator1/1

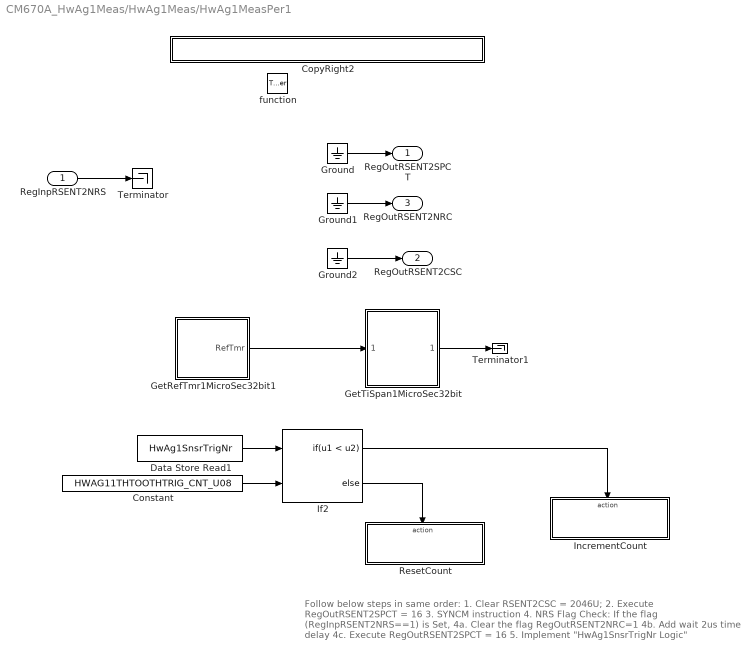
== system CM670A_HwAg1Meas/HwAg1Meas/HwAg1MeasPer1 ==
  note: Follow below steps in same order:
      |
      | 1. Clear RSENT2CSC = 2046U;
      | 2. Execute RegOutRSENT2SPCT = 16
      | 3. SYNCM instruction
      | 4. NRS Flag Check: If the flag (RegInpRSENT2NRS==1) is Set,
      | 	4a. Clear the flag RegOutRSENT2NRC=1
      | 	4b. Add wait 2us time delay
      | 	4c. Execute RegOutRSENT2SPCT = 16
      |
      | 5. Implement "HwAg1SnsrTrigNr Logic"
  RegInpRSENT2NRS : Inport
  function : TriggerPort  TriggerType=function-call
  Constant : Constant  Value=HWAG11THTOOTHTRIG_CNT_U08
      settings: AttributesFormatString=%<Value>.EngVal = 2
  CopyRight2 : Subsystem  Description=|  mask(Copyright Information){none=on}
      | Copyright info block.                                               
      |                                                                     
      | Place copyright information at the top of every subsystem in design.
      mask prompts: none "No parameters"
      mask help: Place copyright information at the top of every subsystem in design.
      mask Display:
      | NxtrConf = 'Nexteer Confidential';
      | 
      | sys = bdroot; %handle for the current model ("system")
      | first = get_param(sys,'Created');
      | first = first(end-3:end);  %year is last four digits
      | 
      | last = get_param(sys,'LastModifiedDate');
      | if isempty(last)
      |     last = datestr(now,'yyyy');
      | else
      |     last = last(end-3:end);
      | end
      | 
      | if strcmp(first,last)
      |     fprintf('%s -- Copyright %s Nexteer',NxtrConf,first)
      | else
      |     fprintf('%s -- %s%s- %s Nexteer',NxtrConf,char(169),first,last)
      | end
  Data Store Read1 : DataStoreRead  DataStoreName=HwAg1SnsrTrigNr
  GetRefTmr1MicroSec32bit1 : Subsystem
      settings: AttributesFormatString=Client Call : Start Time
  GetTiSpan1MicroSec32bit : Subsystem
  Ground : Ground
  Ground1 : Ground
  Ground2 : Ground
  If2 : If  RequirementInfo={} %GIDa_52887fb4_6e2d_4085_a59f_5fb5467e86e8  NumInputs=2  IfExpression=u1 < u2
  IncrementCount : Subsystem  RequirementInfo={} %GIDa_0b671363_7dae_45b8_addf_de184e1c6d89  TreatAsAtomicUnit=on
  ResetCount : Subsystem  RequirementInfo={} %GIDa_82eef91c_2351_41df_bcad_e1b6c9f74967  TreatAsAtomicUnit=on
  Terminator : Terminator
  Terminator1 : Terminator
  RegOutRSENT2SPCT : Outport
  RegOutRSENT2CSC : Outport  Port=2
  RegOutRSENT2NRC : Outport  Port=3
  wires:
  Ground/1 -> RegOutRSENT2SPCT/1
  Ground2/1 -> RegOutRSENT2CSC/1
  RegInpRSENT2NRS/1 -> Terminator/1
  GetTiSpan1MicroSec32bit/1(TiSpan) -> Terminator1/1
  GetRefTmr1MicroSec32bit1/1(RefTmr) -> GetTiSpan1MicroSec32bit/1(RefTmr)
  Ground1/1 -> RegOutRSENT2NRC/1
  If2/1 -> IncrementCount/Action
  If2/2 -> ResetCount/Action
  Data Store Read1/1 -> If2/1
  Constant/1 -> If2/2

== system CM670A_HwAg1Meas/HwAg1Meas/HwAg1MeasPer2 ==
  note: Follow below steps in same order:
      |
      | 1. Check the Sensor Seq Number
      |    1a. Check Sensor Seq Number Logic first
      |    1b. Execute RawHwAgRead
      |    1c. Clear RSENT2CSC = 2046U;
      |    1d. FRS Flag Check: If the RegInpRSENT2FRS==1,  Read the RegInpRSENT2FND
      |
      | Design Note: Registers Read must be done once only. (Pl. see Design Rational Section for detail)
  RegInpRSENT2CS : Inport
  RegInpRSENT2FRXD : Inport  Port=2
  RegInpRSENT2FRS : Inport  Port=3
  RegInpRSENT2FND : Inport  Port=4
  function : TriggerPort  TriggerType=function-call
  Constant : Constant  Value=HWAG10THTOOTHTRIG_CNT_U08
      settings: AttributesFormatString=%<Value>.EngVal = 1
  CopyRight2 : Subsystem  Description=|  mask(Copyright Information){none=on}
      | Copyright info block.                                               
      |                                                                     
      | Place copyright information at the top of every subsystem in design.
      mask prompts: none "No parameters"
      mask help: Place copyright information at the top of every subsystem in design.
      mask Display:
      | NxtrConf = 'Nexteer Confidential';
      | 
      | sys = bdroot; %handle for the current model ("system")
      | first = get_param(sys,'Created');
      | first = first(end-3:end);  %year is last four digits
      | 
      | last = get_param(sys,'LastModifiedDate');
      | if isempty(last)
      |     last = datestr(now,'yyyy');
      | else
      |     last = last(end-3:end);
      | end
      | 
      | if strcmp(first,last)
      |     fprintf('%s -- Copyright %s Nexteer',NxtrConf,first)
      | else
      |     fprintf('%s -- %s%s- %s Nexteer',NxtrConf,char(169),first,last)
      | end
  Data Store Read : DataStoreRead  DataStoreName=HwAg1SnsrTrigNr
  If1 : If  RequirementInfo={} %GIDa_b9d998a2_4248_48bf_b95a_652bbcf823e0  NumInputs=2  IfExpression=u1 == u2
  Merge : Merge
  Merge1 : Merge
  Snsr0Read : Subsystem  RequirementInfo={} %GIDa_2b179ee7_c14d_4158_a836_7aa0dadc399b  TreatAsAtomicUnit=on
  Snsr0Read1 : Subsystem  RequirementInfo={} %GIDa_2e58aaa8_37af_463e_9d00_f3ca0f076d23  TreatAsAtomicUnit=on
  HwAg1Snsr0Raw : Outport
  HwAg1Snsr0TestOk : Outport  Port=2
  wires:
  Data Store Read/1 -> If1/1
  If1/1 -> Snsr0Read/Action
  If1/2 -> Snsr0Read1/Action
  Merge/1 -> HwAg1Snsr0Raw/1
  Merge1/1 -> HwAg1Snsr0TestOk/1
  Snsr0Read/1(HwAg1Snsr0Raw) -> Merge/1
  Snsr0Read1/1(HwAg1Snsr0Raw) -> Merge/2
  Snsr0Read/2(HwAg1Snsr0TestOk) -> Merge1/1
  Snsr0Read1/2(HwAg1Snsr0TestOk) -> Merge1/2
  RegInpRSENT2FRXD/1 -> Snsr0Read/2(RegInpRSENT2FRXD)
  RegInpRSENT2CS/1 -> Snsr0Read/1(RegInpRSENT2CS)
  RegInpRSENT2FRS/1 -> Snsr0Read/3(RegInpRSENT2FRS)
  RegInpRSENT2FND/1 -> Snsr0Read/4(RegInpRSENT2FND)
  Constant/1 -> If1/2
